simulink model "LEGO_DC_Motor"  (R2013b)
settings: Solver=ode3  SolverMode=SingleTasking  StartTime=0.0  StopTime=10.0  RelTol=1e-3
PostLoadFcn:
  | Ts = 0.1;
  | ts1 = 0.004;
  | a_d = 0.8;
InitFcn:
  | Ts = 0.1;
  | ts1 = 0.004;
  | a_d = 0.8;
undefined symbols (not defined in the file or in its folder): sigbuilder_block
libraries: legonxtlib x3, slident x1
CloseFcn:
  | clear Ts ts1 a_d
settings Model: SimulationMode=external  ExtModeTrigDuration=2  Creator=Alphonso Monk  LastModifiedBy=Alphonso Monk
settings OptimizationCC: OptimizeModelRefInitCode=on  LifeSpan=1
settings DebuggingCC: SolverPrmCheckMsg=none
settings HardwareCC: ProdLargestAtomicInteger=Long  ProdLargestAtomicFloat=Float  ProdEndianess=LittleEndian  ProdHWDeviceType=ARM Compatible->ARM 7
settings RTWCC: SystemTargetFile=realtime.tlc  GenerateMakefile=off  TemplateMakefile=realtime.tmf  Description=Run on Target Hardware  RTWVerbose=off  ProcessScript=realtime_make_rtw_hook
settings STFCustomTargetCC: TargetLibSuffix=.a  GenerateSampleERTMain=on  ERTCustomFileBanners=on  SupportNonInlinedSFcns=off  SupportVariableSizeSignals=on  MATLABClassNameForMDSCustomization=Simulink.SoftwareTarget.ERTCustomization  GRTInterface=off  SystemTargetFile=realtime.tlc
settings ERTTargetCC: CodeReplacementLibrary=ANSI_C  GenerateSampleERTMain=on  ParMdlRefBuildCompliant=off  CompOptLevelCompliant=off  ConcurrentExecutionCompliant=off  CombineOutputUpdateFcns=off  ERTFirstTimeCompliant=off  SupportContinuousTime=on  SupportVariableSizeSignals=on  ModelStepFunctionPrototypeControlCompliant=off  CPPClassGenCompliant=off  ExtMode=on  ExtModeTransport=2  ExtModeMexArgs=0 3 9600 30  InlinedParameterPlacement=NonHierarchical  ERTSrcFileBannerTemplate=realtime_code_template.cgt  ERTHdrFileBannerTemplate=realtime_code_template.cgt  ERTDataSrcFileTemplate=realtime_code_template.cgt  ERTDataHdrFileTemplate=realtime_code_template.cgt  ERTCustomFileTemplate=realtime_file_process.tlc

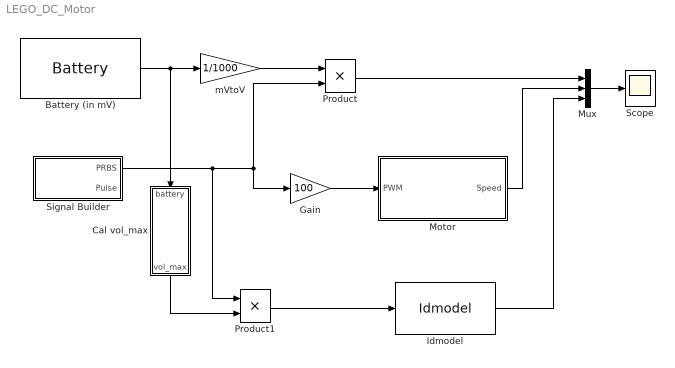
== system LEGO_DC_Motor ==
  Battery (in mV) : legonxtlib/Battery  sampleTime=Ts
  Cal vol_max : Subsystem
  Gain : Gain  Gain=100
  "Idmodel " : slident/Idmodel   sys=sysTF  IC=0  noi=off  seed=[]
  Motor : Subsystem
  Mux : Mux  Inputs=3
  Product : Product  Inputs=**
  Product1 : Product  Inputs=**
  Scope : Scope
      settings: SaveName=motorResponse
  Signal Builder : Subsystem  Tag=STV Subsys  LoadFcn=sigbuilder_block('load');  StartFcn=sigbuilder_block('start');  StopFcn=sigbuilder_block('stop');  ClipboardFcn=sigbuilder_block('clipboard');  mask(Sigbuilder block){}
      mask help: Simulink:masks:SigbuilderBlock_MD
      mask init:
      | if ~strcmp(get_param(bdroot(gcbh),'SimulationStatus'),'stopped') tuvar = sigbuilder_block('maskInit'); end
      settings: CopyFcn=sigbuilder_block('copy');  DeleteFcn=sigbuilder_block('delete');  ModelCloseFcn=sigbuilder_block('modelClose');  PreSaveFcn=sigbuilder_block('preSave');  PauseFcn=sigbuilder_block('pause');  ContinueFcn=sigbuilder_block('continue');  NameChangeFcn=sigbuilder_block('namechange');  OpenFcn=sigbuilder_block('open',[0 30 1020 489 ]);  CloseFcn=sigbuilder_block('close');
      mask Display: plot(0, 0, 100, 100,[2, 2, 32, 32, 2], [68, 8, 8, 68, 68],[32, 2], [38, 38], [32, 19, 2],[53, 60, 44], [32, 17, 17, 2],[16, 16, 31, 31]);txt = getActiveGroup(gcbh);text(2, 100, txt,'verticalAlignment', 'top');
  mVtoV : Gain  Gain=1/1000
  wires:
  Product/1 -> Mux/1
  Mux/1 -> Scope/1
  Motor/1(Speed) -> Mux/2
  mVtoV/1 -> Product/1
  Signal Builder/1(PRBS) -> Product1/1, Product/2, Gain/1
  Gain/1 -> Motor/1(PWM)
  "Idmodel "/1 -> Mux/3
  Battery (in mV)/1 -> mVtoV/1, Cal vol_max/1(battery)
  Product1/1 -> "Idmodel "/1
  Cal vol_max/1(vol_max) -> Product1/2

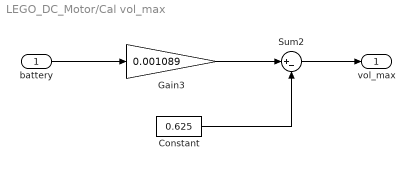
== system LEGO_DC_Motor/Cal vol_max ==
  battery : Inport
  Constant : Constant  Value=0.625  OutDataTypeStr=single
      settings: AttributesFormatString=DataType = %<OutDataTypeStr>
  Gain3 : Gain  Gain=0.001089  OutDataTypeStr=Inherit: Same as input  ParamDataTypeStr=Inherit: Same as input
  Sum2 : Sum  Inputs=|+-  OutDataTypeStr=Inherit: Same as first input
  vol_max : Outport
  wires:
  Gain3/1 -> Sum2/1
  Sum2/1 -> vol_max/1
  Constant/1 -> Sum2/2
  battery/1 -> Gain3/1

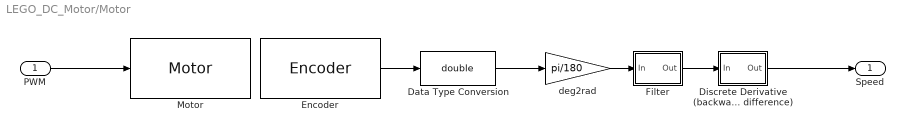
== system LEGO_DC_Motor/Motor ==
  PWM : Inport
  Data Type Conversion : DataTypeConversion  OutDataTypeStr=double
  Discrete Derivative (backward difference) : Subsystem
  Encoder : legonxtlib/Encoder  portNumber=B  opMode=No reset  sampleTime=ts1
  Filter : Subsystem
  Motor : legonxtlib/Motor  sportNumber=B  sstopAction=Brake
  deg2rad : Gain  Gain=pi/180  OutDataTypeStr=Inherit: Same as input  ParamDataTypeStr=Inherit: Same as input
  Speed : Outport
  wires:
  Discrete Derivative (backward difference)/1(Out) -> Speed/1
  PWM/1 -> Motor/1
  Filter/1(Out) -> Discrete Derivative (backward difference)/1(In)
  deg2rad/1 -> Filter/1(In)
  Data Type Conversion/1 -> deg2rad/1
  Encoder/1 -> Data Type Conversion/1

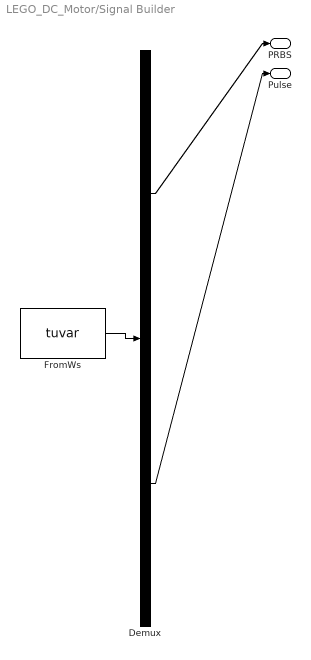
== system LEGO_DC_Motor/Signal Builder ==
  Demux : Demux  Tag=STV Demux  Outputs=2
  FromWs : FromWorkspace  Tag=STV FromWs  VariableName=tuvar  SampleTime=0
      SigBuilderData=|
      | common.afterFinalStr = 'Extrapolate'
      | common.sampleTime = 0
      | dataSet.timeRange = [0 100]
      | dataSet.name = 'SysIdent'
      | sbobj.Groups.Name = 'SysIdent'
      | sbobj.Groups.Signals(1).Name = 'PRBS'
      | sbobj.Groups.Signals(1).XData = [0 2 2 8 8 10 10 14 14 16 16 18 18 22 22 30 30 32 32 42 42 44 44 46 46 48 48 50 50 58 58 62 62 64 64 66 66 72 72 76 76 82 82 88 88 90 90 94 94 100]
      | sbobj.Groups.Signals(1).YData = [-1 -1 1 1 -1 -1 1 1 -1 -1 1 1 -1 -1 1 1 -1 -1 1 1 -1 -1 1 1 -1 -1 1 1 -1 -1 1 1 -1 -1 1 1 -1 -1 1 1 -1 -1 1 1 -1 -1 1 1 -1 -1]
      | sbobj.Groups.Signals(2).Name = 'Pulse'
      | sbobj.Groups.Signals(2).XData = [0 4 4 6 6 100]
      | sbobj.Groups.Signals(2).YData = [0 0 100 100 0 0]
      | sbobj.Groups.TimeRange = [0 100]
  PRBS : Outport  Tag=STV Outport
  Pulse : Outport  Tag=STV Outport  Port=2
  wires:
  FromWs/1 -> Demux/1
  Demux/1 -> PRBS/1
  Demux/2 -> Pulse/1

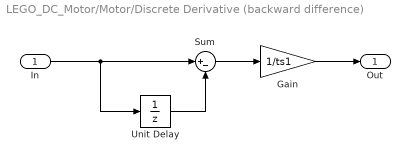
== system LEGO_DC_Motor/Motor/Discrete Derivative (backward difference) ==
  In : Inport
  Gain : Gain  Gain=1/ts1  OutDataTypeStr=Inherit: Same as input  ParamDataTypeStr=Inherit: Same as input
  Sum : Sum  Inputs=|+-  OutDataTypeStr=Inherit: Same as first input
  Unit Delay : UnitDelay  SampleTime=-1
  Out : Outport
  wires:
  Gain/1 -> Out/1
  In/1 -> Sum/1, Unit Delay/1
  Unit Delay/1 -> Sum/2
  Sum/1 -> Gain/1

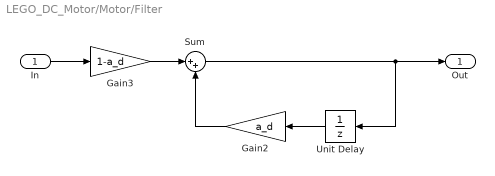
== system LEGO_DC_Motor/Motor/Filter ==
  In : Inport
  Gain2 : Gain  Gain=a_d  OutDataTypeStr=Inherit: Same as input  ParamDataTypeStr=Inherit: Same as input
  Gain3 : Gain  Gain=1-a_d  OutDataTypeStr=Inherit: Same as input  ParamDataTypeStr=Inherit: Same as input
  Sum : Sum  Inputs=|++  OutDataTypeStr=Inherit: Same as first input
  Unit Delay : UnitDelay  SampleTime=-1
  Out : Outport
  wires:
  In/1 -> Gain3/1
  Gain3/1 -> Sum/1
  Gain2/1 -> Sum/2
  Unit Delay/1 -> Gain2/1
  Sum/1 -> Out/1, Unit Delay/1
